simulink model "Linear_model_Kalman_Bucy"  (R2025b)
settings: Solver=VariableStepAuto  StartTime=0.0  StopTime=10.0  RelTol=1e-3
values from neighbouring files (symbols this model uses):
  A1 = [0, 1; 0, 0]    [Q5_7_kalman_observer_linear.m]
  A2 = [0, 0, 1, 0; 0, 0, 0, 1; 0, g, 0, 0; 0, 0, 0, 0]    [Q5_7_kalman_observer_linear.m]
  A3 = [0, 0, 1, 0; 0, 0, 0, 1; 0, -g, 0, 0; 0, 0, 0, 0]    [Q5_7_kalman_observer_linear.m]
  A4 = [0, 1; 0, 0]    [Q5_7_kalman_observer_linear.m]
  B1 = [0; 1/m]    [Q5_7_kalman_observer_linear.m]
  B2 = [0; 0; 0; 1/J11]    [Q5_7_kalman_observer_linear.m]
  B3 = [0; 0; 0; 1/J22]    [Q5_7_kalman_observer_linear.m]
  B4 = [0; 1/J33]    [Q5_7_kalman_observer_linear.m]
  C1 = eye(2)    [Q5_7_kalman_observer_linear.m]
  C2 = eye(4)    [Q5_7_kalman_observer_linear.m]
  C3 = eye(4)    [Q5_7_kalman_observer_linear.m]
  C4 = eye(2)    [Q5_7_kalman_observer_linear.m]
  D1 = zeros(2, 1)    [Q5_7_kalman_observer_linear.m]
  D2 = zeros(4, 1)    [Q5_7_kalman_observer_linear.m]
  D3 = zeros(4, 1)    [Q5_7_kalman_observer_linear.m]
  D4 = zeros(2, 1)    [Q5_7_kalman_observer_linear.m]
  K1 = place(A1, B1, poles1)    [Q5_7_kalman_observer_linear.m]
  K2 = place(A2, B2, poles2)    [Q5_7_kalman_observer_linear.m]
  K3 = place(A3, B3, poles3)    [Q5_7_kalman_observer_linear.m]
  K4 = place(A4, B4, poles4)    [Q5_7_kalman_observer_linear.m]
  ki1 = prefilter(A1, B1, C1(1,:), K1)    [Q5_7_kalman_observer_linear.m]
  ki2 = prefilter(A2, B2, C2(1,:), K2)    [Q5_7_kalman_observer_linear.m]
  ki3 = prefilter(A3, B3, C3(1,:), K3)    [Q5_7_kalman_observer_linear.m]
  ki4 = prefilter(A4, B4, C4(1,:), K4)    [Q5_7_kalman_observer_linear.m]
  noise_P_lat = [var_P_r2,  var_P_th1, var_P_v2,  var_P_om1] * Ts    [Q5_7_kalman_observer_linear.m]
  noise_P_lon = [var_P_r1,  var_P_th2, var_P_v1,  var_P_om2] * Ts    [Q5_7_kalman_observer_linear.m]
  noise_P_vert = [var_P_r3,  var_P_v3]                         * Ts    [Q5_7_kalman_observer_linear.m]
  noise_P_yaw = [var_P_th3, var_P_om3]                        * Ts    [Q5_7_kalman_observer_linear.m]
  phi_ref = 0.5    [Q5_7_kalman_observer_linear.m]
  R0_lat_k = R0_lat    [Q5_7_kalman_observer_linear.m]
  R0_lon_k = R0_lon    [Q5_7_kalman_observer_linear.m]
  R0_vert_k = R0_vert    [Q5_7_kalman_observer_linear.m]
  R0_yaw_k = R0_yaw    [Q5_7_kalman_observer_linear.m]
  Ts = 0.01    [Q5_7_kalman_observer_linear.m]
  x0_1 = [0; 0]    [Q5_7_kalman_observer_linear.m]
  x0_2 = [0; 0; 0; 0]    [Q5_7_kalman_observer_linear.m]
  x0_3 = [0; 0; 0; 0]    [Q5_7_kalman_observer_linear.m]
  x0_4 = [0; 0]    [Q5_7_kalman_observer_linear.m]
  x0_obs1 = [3; 0]    [Q5_7_kalman_observer_linear.m]
  x0_obs2 = [3; 0; 0; 0]    [Q5_7_kalman_observer_linear.m]
  x0_obs3 = [3; 0; 0; 0]    [Q5_7_kalman_observer_linear.m]
  x0_obs4 = [0.5; 0]    [Q5_7_kalman_observer_linear.m]
  x_ref = 2    [Q5_7_kalman_observer_linear.m]
  y_ref = 1    [Q5_7_kalman_observer_linear.m]
  z_ref = 4    [Q5_7_kalman_observer_linear.m]
undefined symbols (not defined in the file or in its folder): Continuous, Time
libraries: simulink x8, ctrlSharedLib x4
settings Model: Creator=joaom  LastModifiedBy=pepev
settings DataIOCC: SaveFormat=Array

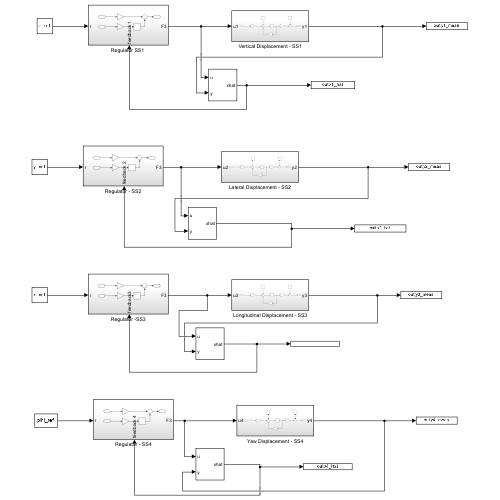
[thumbnail: Simulink's stored preview of the top-level diagram]
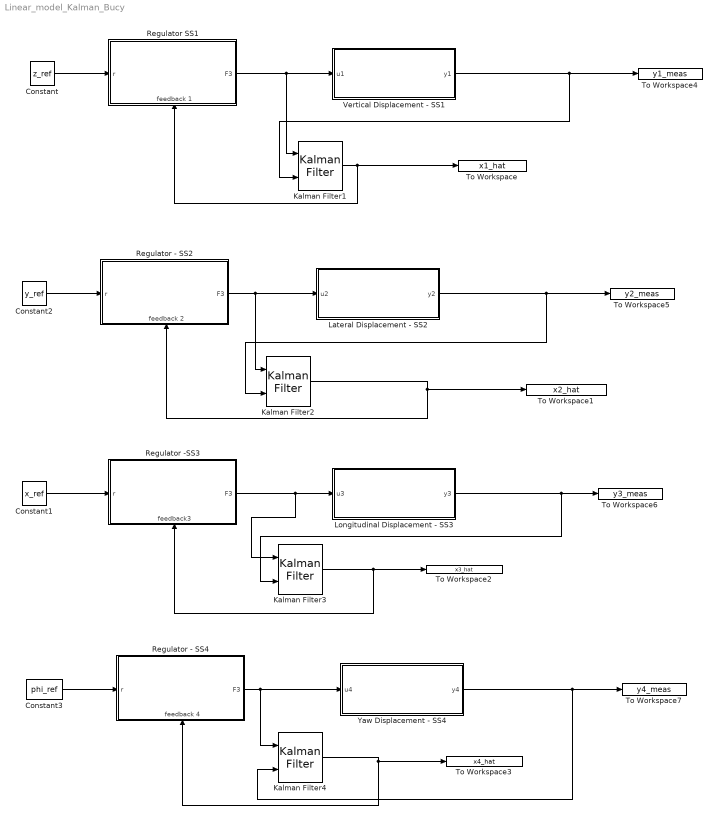
== system Linear_model_Kalman_Bucy ==
  Constant : Constant  Value=z_ref
  Constant1 : Constant  Value=x_ref
  Constant2 : Constant  Value=y_ref
  Constant3 : Constant  Value=phi_ref
  Kalman Filter1 : ctrlSharedLib/Kalman Filter  TimeDomain=Continuous-Time  UseCurrentEstimator=on  ModelSource=LTI State-Space Variable  ModelSourceVariable=ss(A1,B1,C1,D1)  A=0.95  B=1  C=1  D=0  NumberOfStates=1  NumberOfInputs=1  NumberOfOutputs=1  InitialEstimateSource=Dialog  X0=x0_obs1  P0=10  UseK=off  UseGH=off  NumberOfProcessNoiseInputs=1  G=1  TimeInvariantG=on  H=0  TimeInvariantH=on  Q=Q0_vert_k  TimeInvariantQ=on  R=R0_vert_k  TimeInvariantR=on  N=0  TimeInvariantN=on  AddInputPort=on  AddEnablePort=off  OutputEstimatedY=off  OutputP=off  Ts=-1
  Kalman Filter2 : ctrlSharedLib/Kalman Filter  TimeDomain=Continuous-Time  UseCurrentEstimator=on  ModelSource=LTI State-Space Variable  ModelSourceVariable=ss(A2,B2,C2,D2)  A=0.95  B=1  C=1  D=0  NumberOfStates=1  NumberOfInputs=1  NumberOfOutputs=1  InitialEstimateSource=Dialog  X0=x0_obs2  P0=10  UseK=off  UseGH=off  NumberOfProcessNoiseInputs=1  G=1  TimeInvariantG=on  H=0  TimeInvariantH=on  Q=Q0_lat_k  TimeInvariantQ=on  R=R0_lat_k  TimeInvariantR=on  N=0  TimeInvariantN=on  AddInputPort=on  AddEnablePort=off  OutputEstimatedY=off  OutputP=off  Ts=-1
  Kalman Filter3 : ctrlSharedLib/Kalman Filter  TimeDomain=Continuous-Time  UseCurrentEstimator=on  ModelSource=LTI State-Space Variable  ModelSourceVariable=ss(A3,B3,C3,D3)  A=0.95  B=1  C=1  D=0  NumberOfStates=1  NumberOfInputs=1  NumberOfOutputs=1  InitialEstimateSource=Dialog  X0=x0_obs3  P0=10  UseK=off  UseGH=off  NumberOfProcessNoiseInputs=1  G=1  TimeInvariantG=on  H=0  TimeInvariantH=on  Q=Q0_lon_k  TimeInvariantQ=on  R=R0_lon_k  TimeInvariantR=on  N=0  TimeInvariantN=on  AddInputPort=on  AddEnablePort=off  OutputEstimatedY=off  OutputP=off  Ts=-1
  Kalman Filter4 : ctrlSharedLib/Kalman Filter  TimeDomain=Continuous-Time  UseCurrentEstimator=on  ModelSource=LTI State-Space Variable  ModelSourceVariable=ss(A4,B4,C4,D4)  A=0.95  B=1  C=1  D=0  NumberOfStates=1  NumberOfInputs=1  NumberOfOutputs=1  InitialEstimateSource=Dialog  X0=x0_obs4  P0=10  UseK=off  UseGH=off  NumberOfProcessNoiseInputs=1  G=1  TimeInvariantG=on  H=0  TimeInvariantH=on  Q=Q0_yaw_k  TimeInvariantQ=on  R=R0_yaw_k  TimeInvariantR=on  N=0  TimeInvariantN=on  AddInputPort=on  AddEnablePort=off  OutputEstimatedY=off  OutputP=off  Ts=-1
  Lateral Displacement - SS2 : Subsystem
  Longitudinal Displacement - SS3 : Subsystem
  Regulator - SS2 : Subsystem
      settings: PortSchema="{\"entries\":[{\"content\":{\"sides\":[{\"content\":{\"connectorIds\":[\"In1\"]},\"type\":\"ConnectorPlacement.EquallySpacedRectSide\",\"uuid\":\"b3654a7f-5063-48c0-9b36-91e0db63b0ba\"},{\"content\":{\"connectorIds\":[\"Out1\"],\"side\":\"RIGHT\"},\"type\":\"ConnectorPlacement.EquallySpacedRectSide\",\"uuid\":\"218488d6-68f2-41aa-8299-f3fb09ba40d8\"},{\"content\":{\"side\":\"TOP\"},\"type\":\"ConnectorPlacement.EquallySpacedRectSide\",\"uuid\":\"ffca8f5f-99ce-4cfe-b848-505d5918397a\"},{\"content\":{\"connectorIds\":[\"In2\"],\"side\":\"BOTTOM\"},\"type\":\"ConnectorPlacement.EquallySpacedRectSide\",\"uuid\":\"0ee1b0b7-fa1d-4d2f-b721-1db90edeb8b7\"}]},\"type\":\"ConnectorPlacement.EquallySpacedConnector\",\"uuid\":\"97e1b17e-acc2-4e54-bcf8-8316abbe6834\"}],\"packageUris\":[\"http://schema.mathworks.com/mf0/Connector/R2020b\"],\"version\":\"1.0\"}"
  Regulator - SS4 : Subsystem
      settings: PortSchema="{\"entries\":[{\"content\":{\"sides\":[{\"content\":{\"connectorIds\":[\"In1\"]},\"type\":\"ConnectorPlacement.EquallySpacedRectSide\",\"uuid\":\"b3654a7f-5063-48c0-9b36-91e0db63b0ba\"},{\"content\":{\"connectorIds\":[\"Out1\"],\"side\":\"RIGHT\"},\"type\":\"ConnectorPlacement.EquallySpacedRectSide\",\"uuid\":\"218488d6-68f2-41aa-8299-f3fb09ba40d8\"},{\"content\":{\"side\":\"TOP\"},\"type\":\"ConnectorPlacement.EquallySpacedRectSide\",\"uuid\":\"ffca8f5f-99ce-4cfe-b848-505d5918397a\"},{\"content\":{\"connectorIds\":[\"In2\"],\"side\":\"BOTTOM\"},\"type\":\"ConnectorPlacement.EquallySpacedRectSide\",\"uuid\":\"0ee1b0b7-fa1d-4d2f-b721-1db90edeb8b7\"}]},\"type\":\"ConnectorPlacement.EquallySpacedConnector\",\"uuid\":\"97e1b17e-acc2-4e54-bcf8-8316abbe6834\"}],\"packageUris\":[\"http://schema.mathworks.com/mf0/Connector/R2020b\"],\"version\":\"1.0\"}"
  Regulator -SS3 : Subsystem
      settings: PortSchema="{\"entries\":[{\"content\":{\"sides\":[{\"content\":{\"connectorIds\":[\"In1\"]},\"type\":\"ConnectorPlacement.EquallySpacedRectSide\",\"uuid\":\"b3654a7f-5063-48c0-9b36-91e0db63b0ba\"},{\"content\":{\"connectorIds\":[\"Out1\"],\"side\":\"RIGHT\"},\"type\":\"ConnectorPlacement.EquallySpacedRectSide\",\"uuid\":\"218488d6-68f2-41aa-8299-f3fb09ba40d8\"},{\"content\":{\"side\":\"TOP\"},\"type\":\"ConnectorPlacement.EquallySpacedRectSide\",\"uuid\":\"ffca8f5f-99ce-4cfe-b848-505d5918397a\"},{\"content\":{\"connectorIds\":[\"In2\"],\"side\":\"BOTTOM\"},\"type\":\"ConnectorPlacement.EquallySpacedRectSide\",\"uuid\":\"0ee1b0b7-fa1d-4d2f-b721-1db90edeb8b7\"}]},\"type\":\"ConnectorPlacement.EquallySpacedConnector\",\"uuid\":\"97e1b17e-acc2-4e54-bcf8-8316abbe6834\"}],\"packageUris\":[\"http://schema.mathworks.com/mf0/Connector/R2020b\"],\"version\":\"1.0\"}"
  "Regulator SS1 " : Subsystem
      settings: PortSchema="{\"entries\":[{\"content\":{\"sides\":[{\"content\":{\"connectorIds\":[\"In1\"]},\"type\":\"ConnectorPlacement.EquallySpacedRectSide\",\"uuid\":\"b3654a7f-5063-48c0-9b36-91e0db63b0ba\"},{\"content\":{\"connectorIds\":[\"Out1\"],\"side\":\"RIGHT\"},\"type\":\"ConnectorPlacement.EquallySpacedRectSide\",\"uuid\":\"218488d6-68f2-41aa-8299-f3fb09ba40d8\"},{\"content\":{\"side\":\"TOP\"},\"type\":\"ConnectorPlacement.EquallySpacedRectSide\",\"uuid\":\"ffca8f5f-99ce-4cfe-b848-505d5918397a\"},{\"content\":{\"connectorIds\":[\"In2\"],\"side\":\"BOTTOM\"},\"type\":\"ConnectorPlacement.EquallySpacedRectSide\",\"uuid\":\"0ee1b0b7-fa1d-4d2f-b721-1db90edeb8b7\"}]},\"type\":\"ConnectorPlacement.EquallySpacedConnector\",\"uuid\":\"97e1b17e-acc2-4e54-bcf8-8316abbe6834\"}],\"packageUris\":[\"http://schema.mathworks.com/mf0/Connector/R2020b\"],\"version\":\"1.0\"}"
  To Workspace : ToWorkspace  VariableName=x1_hat  SampleTime=-1
  To Workspace1 : ToWorkspace  VariableName=x2_hat  SampleTime=-1
  To Workspace2 : ToWorkspace  VariableName=x3_hat  SampleTime=-1
  To Workspace3 : ToWorkspace  VariableName=x4_hat  SampleTime=-1
  To Workspace4 : ToWorkspace  VariableName=y1_meas  SampleTime=-1
  To Workspace5 : ToWorkspace  VariableName=y2_meas  SampleTime=-1
  To Workspace6 : ToWorkspace  VariableName=y3_meas  SampleTime=-1
  To Workspace7 : ToWorkspace  VariableName=y4_meas  SampleTime=-1
  Vertical Displacement - SS1 : Subsystem
  Yaw Displacement - SS4 : Subsystem
  wires:
  Constant/1 -> "Regulator SS1 "/1(r)
  "Regulator SS1 "/1(F3) -> Kalman Filter1/1, Vertical Displacement - SS1/1(u1)
  Constant2/1 -> Regulator - SS2/1(r)
  Regulator - SS2/1(F3) -> Kalman Filter2/1, Lateral Displacement - SS2/1(u2)
  Constant1/1 -> Regulator -SS3/1(r)
  Regulator -SS3/1(F3) -> Kalman Filter3/1, Longitudinal Displacement - SS3/1(u3)
  Yaw Displacement - SS4/1(y4) -> To Workspace7/1, Kalman Filter4/2
  Constant3/1 -> Regulator - SS4/1(r)
  Regulator - SS4/1(F3) -> Yaw Displacement - SS4/1(u4), Kalman Filter4/1
  Kalman Filter1/1 -> To Workspace/1, "Regulator SS1 "/2(feedback 1)
  Kalman Filter3/1 -> Regulator -SS3/2(feedback3), To Workspace2/1
  Kalman Filter4/1 -> To Workspace3/1, Regulator - SS4/2(feedback 4)
  Kalman Filter2/1 -> Regulator - SS2/2(feedback 2), To Workspace1/1
  Vertical Displacement - SS1/1(y1) -> To Workspace4/1, Kalman Filter1/2
  Lateral Displacement - SS2/1(y2) -> To Workspace5/1, Kalman Filter2/2
  Longitudinal Displacement - SS3/1(y3) -> To Workspace6/1, Kalman Filter3/2

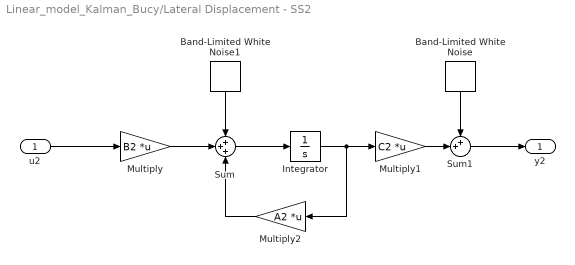
== system Linear_model_Kalman_Bucy/Lateral Displacement - SS2 ==
  u2 : Inport
  Band-Limited White Noise : simulink/Sources/Band-Limited White Noise  Cov=noise_M_lat  Ts=0.01  seed=[50 51 52 53]
  Band-Limited White Noise1 : simulink/Sources/Band-Limited White Noise  Cov=[noise_P_lat]  Ts=0.01  seed=[46 47 48 49]
  Integrator : Integrator  InitialCondition=x0_2
  Multiply : Gain  Gain=B2  Multiplication=Matrix(K*u)
  Multiply1 : Gain  Gain=C2  Multiplication=Matrix(K*u)
  Multiply2 : Gain  Gain=A2  Multiplication=Matrix(K*u)
  Sum : Sum  Inputs=+++
  Sum1 : Sum  Inputs=++|
  y2 : Outport
  wires:
  u2/1 -> Multiply/1
  Multiply/1 -> Sum/2
  Sum/1 -> Integrator/1
  Integrator/1 -> Multiply2/1, Multiply1/1
  Multiply1/1 -> Sum1/2
  Sum1/1 -> y2/1
  Multiply2/1 -> Sum/3
  Band-Limited White Noise/1 -> Sum1/1
  Band-Limited White Noise1/1 -> Sum/1

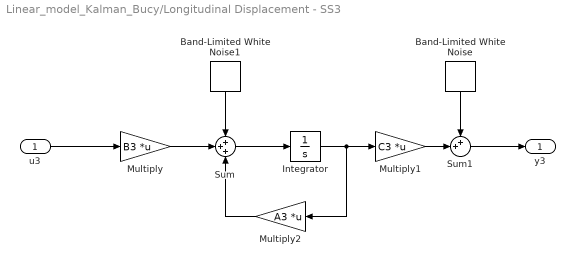
== system Linear_model_Kalman_Bucy/Longitudinal Displacement - SS3 ==
  u3 : Inport
  Band-Limited White Noise : simulink/Sources/Band-Limited White Noise  Cov=noise_M_lon  Ts=0.01  seed=[58 59 60 61]
  Band-Limited White Noise1 : simulink/Sources/Band-Limited White Noise  Cov=[noise_P_lon]  Ts=0.01  seed=[54 55 56 57]
  Integrator : Integrator  InitialCondition=x0_3
  Multiply : Gain  Gain=B3  Multiplication=Matrix(K*u)
  Multiply1 : Gain  Gain=C3  Multiplication=Matrix(K*u)
  Multiply2 : Gain  Gain=A3  Multiplication=Matrix(K*u)
  Sum : Sum  Inputs=+++
  Sum1 : Sum  Inputs=++|
  y3 : Outport
  wires:
  u3/1 -> Multiply/1
  Multiply/1 -> Sum/2
  Sum/1 -> Integrator/1
  Integrator/1 -> Multiply2/1, Multiply1/1
  Multiply1/1 -> Sum1/2
  Sum1/1 -> y3/1
  Multiply2/1 -> Sum/3
  Band-Limited White Noise/1 -> Sum1/1
  Band-Limited White Noise1/1 -> Sum/1

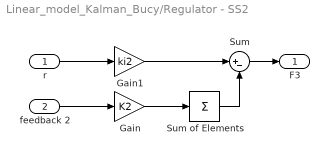
== system Linear_model_Kalman_Bucy/Regulator - SS2 ==
  r : Inport
  feedback 2 : Inport  Port=2
  Gain : Gain  Gain=K2
  Gain1 : Gain  Gain=ki2
  Sum : Sum  Inputs=|+-
  Sum of Elements : Sum  Inputs=+
  F3 : Outport
  wires:
  r/1 -> Gain1/1
  Gain1/1 -> Sum/1
  Sum/1 -> F3/1
  feedback 2/1 -> Gain/1
  Gain/1 -> Sum of Elements/1
  Sum of Elements/1 -> Sum/2

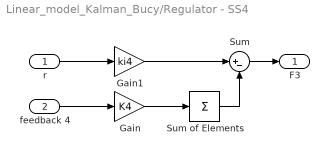
== system Linear_model_Kalman_Bucy/Regulator - SS4 ==
  r : Inport
  feedback 4 : Inport  Port=2
  Gain : Gain  Gain=K4
  Gain1 : Gain  Gain=ki4
  Sum : Sum  Inputs=|+-
  Sum of Elements : Sum  Inputs=+
  F3 : Outport
  wires:
  r/1 -> Gain1/1
  Gain1/1 -> Sum/1
  Sum/1 -> F3/1
  feedback 4/1 -> Gain/1
  Gain/1 -> Sum of Elements/1
  Sum of Elements/1 -> Sum/2

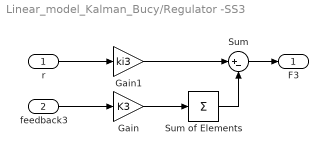
== system Linear_model_Kalman_Bucy/Regulator -SS3 ==
  r : Inport
  feedback3 : Inport  Port=2
  Gain : Gain  Gain=K3
  Gain1 : Gain  Gain=ki3
  Sum : Sum  Inputs=|+-
  Sum of Elements : Sum  Inputs=+
  F3 : Outport
  wires:
  r/1 -> Gain1/1
  Gain1/1 -> Sum/1
  Sum/1 -> F3/1
  feedback3/1 -> Gain/1
  Gain/1 -> Sum of Elements/1
  Sum of Elements/1 -> Sum/2

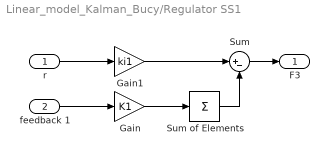
== system Linear_model_Kalman_Bucy/Regulator SS1  ==
  r : Inport
  feedback 1 : Inport  Port=2
  Gain : Gain  Gain=K1
  Gain1 : Gain  Gain=ki1
  Sum : Sum  Inputs=|+-
  Sum of Elements : Sum  Inputs=+
  F3 : Outport
  wires:
  r/1 -> Gain1/1
  Gain1/1 -> Sum/1
  Sum/1 -> F3/1
  feedback 1/1 -> Gain/1
  Gain/1 -> Sum of Elements/1
  Sum of Elements/1 -> Sum/2

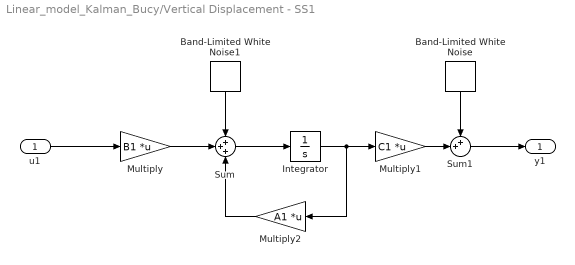
== system Linear_model_Kalman_Bucy/Vertical Displacement - SS1 ==
  u1 : Inport
  Band-Limited White Noise : simulink/Sources/Band-Limited White Noise  Cov=noise_M_vert  Ts=0.01  seed=[44 45]
  Band-Limited White Noise1 : simulink/Sources/Band-Limited White Noise  Cov=[noise_P_vert]  Ts=Ts  seed=[42 43]
  Integrator : Integrator  InitialCondition=x0_1
  Multiply : Gain  Gain=B1  Multiplication=Matrix(K*u)
  Multiply1 : Gain  Gain=C1  Multiplication=Matrix(K*u)
  Multiply2 : Gain  Gain=A1  Multiplication=Matrix(K*u)
  Sum : Sum  Inputs=+++
  Sum1 : Sum  Inputs=++|
  y1 : Outport
  wires:
  u1/1 -> Multiply/1
  Multiply/1 -> Sum/2
  Sum/1 -> Integrator/1
  Integrator/1 -> Multiply2/1, Multiply1/1
  Multiply1/1 -> Sum1/2
  Sum1/1 -> y1/1
  Multiply2/1 -> Sum/3
  Band-Limited White Noise/1 -> Sum1/1
  Band-Limited White Noise1/1 -> Sum/1

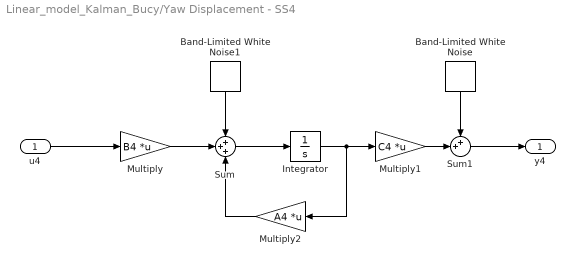
== system Linear_model_Kalman_Bucy/Yaw Displacement - SS4 ==
  u4 : Inport
  Band-Limited White Noise : simulink/Sources/Band-Limited White Noise  Cov=noise_M_yaw  Ts=0.01  seed=[64 65]
  Band-Limited White Noise1 : simulink/Sources/Band-Limited White Noise  Cov=[noise_P_yaw]  Ts=0.01  seed=[62 63]
  Integrator : Integrator  InitialCondition=x0_4
  Multiply : Gain  Gain=B4  Multiplication=Matrix(K*u)
  Multiply1 : Gain  Gain=C4  Multiplication=Matrix(K*u)
  Multiply2 : Gain  Gain=A4  Multiplication=Matrix(K*u)
  Sum : Sum  Inputs=+++
  Sum1 : Sum  Inputs=++|
  y4 : Outport
  wires:
  u4/1 -> Multiply/1
  Multiply/1 -> Sum/2
  Sum/1 -> Integrator/1
  Integrator/1 -> Multiply2/1, Multiply1/1
  Multiply1/1 -> Sum1/2
  Sum1/1 -> y4/1
  Multiply2/1 -> Sum/3
  Band-Limited White Noise/1 -> Sum1/1
  Band-Limited White Noise1/1 -> Sum/1
